simulink model "sitlab7cmain"  (R2018b)
settings: Solver=VariableStepAuto  StartTime=0.0  StopTime=10.0  RelTol=1e-3
settings Model: Creator=student  LastModifiedBy=student

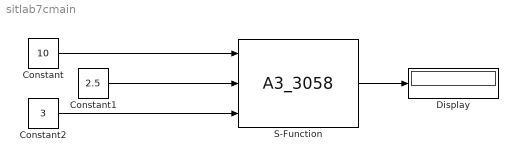
== system sitlab7cmain ==
  Constant : Constant  Value=10
  Constant1 : Constant  Value=2.5
  Constant2 : Constant  Value=3
  Display : Display
  S-Function : S-Function  FunctionName=A3_3058  SFunctionDeploymentMode=off  EnableBusSupport=off
  wires:
  S-Function/1 -> Display/1
  Constant/1 -> S-Function/1
  Constant1/1 -> S-Function/2
  Constant2/1 -> S-Function/3
